simulink model "p3Sim"  (R2020a)
settings: Solver=ode3  StartTime=0.0  StopTime=simPrm.tEnd  FixedStep=simPrm.dt  RelTol=1e-3
values from neighbouring files (symbols this model uses):
  D = D1*D2*D3    [p3Setup.m]
  g = tf(Kc*50*[1 4],[1 10 49 150 0])    [p3Setup.m]
  H = tf(1,[Tau 1])    [p3Setup.m]
undefined symbols (not defined in the file or in its folder): Input
settings Model: Creator=vmali  LastModifiedBy=vmali

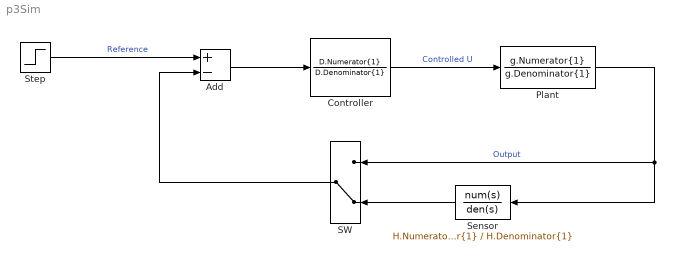
== system p3Sim ==
  Add : Sum  Inputs=+-
  Controller : TransferFcn  Numerator=D.Numerator{1}  Denominator=D.Denominator{1}
  Plant : TransferFcn  Numerator=g.Numerator{1}  Denominator=g.Denominator{1}
  SW : ManualSwitch  CurrentSetting=0
  Sensor : TransferFcn  Numerator=H.Numerator{1}  Denominator=H.Denominator{1}
  Step : Step  Time=Input.Ts  After=Input.A  SampleTime=0
  wires:
  Add/1 -> Controller/1
  Step/1 -> Add/1  "Reference"
  Controller/1 -> Plant/1  "Controlled U"
  Plant/1 -> SW/1, Sensor/1  "Output"
  SW/1 -> Add/2
  Sensor/1 -> SW/2
